simulink subsystem "serial_input_subsystem"  (R2020a)
settings: Solver=VariableStepAuto  StartTime=0.0  StopTime=10.0  RelTol=1e-3
libraries: frdmk64flib x2
settings Model: Creator=Ethan  LastModifiedBy=Ethan

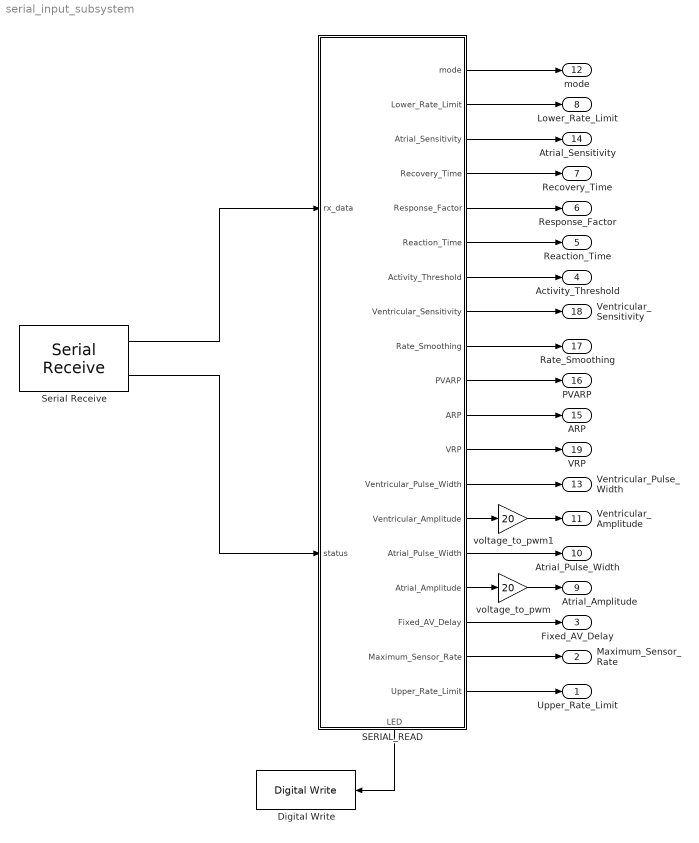
== system serial_input_subsystem ==
  Digital Write : frdmk64flib/Digital Write  Whichpin=BLUE_LED
  SERIAL_READ : Stateflow chart  TreatAsAtomicUnit=on
      settings: PortSchema="{\"entries\":[{\"content\":{\"sides\":[{\"content\":{\"connectorIds\":[\"In2\",\"In1\"]},\"type\":\"ConnectorPlacement.EquallySpacedRectSide\",\"uuid\":\"7925fb1d-c012-46b4-a76b-df094bb3995e\"},{\"content\":{\"connectorIds\":[\"Out1\",\"Out2\",\"Out3\",\"Out4\",\"Out5\",\"Out6\",\"Out7\",\"Out8\",\"Out9\",\"Out10\",\"Out11\",\"Out12\",\"Out13\",\"Out14\",\"Out15\",\"Out16\",\"Out18\",\"Out20\",\"Out19\"],\"side\":\"RIGHT\"},\"type\":\"ConnectorPlacement.EquallySpacedRectSide\",\"uuid\":\"8182b149-1b25-42ed-a9c6-d652f0475bdf\"},{\"content\":{\"connectorIds\":[\"Out17\"],\"side\":\"TOP\"},\"type\":\"ConnectorPlacement.EquallySpacedRectSide\",\"uuid\":\"014ecb25-725b-45bf-b2bd-0487c3cb83c8\"}]},\"type\":\"ConnectorPlacement.EquallySpacedConnector\",\"uuid\":\"b7c7ca09-4347-41ae-aa03-be4e7decd789\"}],\"packageUris\":[\"http://schema.mathworks.com/mf0/Connector/19700101\"],\"version\":\"1.0\"}"
  Serial Receive : frdmk64flib/Serial Receive  SCIModule=0  Baudrate=uint32(9600)  Parity=None  StopBits=1  HardwareFlowControl=None  ByteOrder=LittleEndian  DataType=uint8  DataLength=66  BlockingMode=off  OutputStatus=on  SampleTime=-1
  voltage_to_pwm : Gain  Gain=20  OutDataTypeStr=Inherit: Same as input
  voltage_to_pwm1 : Gain  Gain=20  OutDataTypeStr=Inherit: Same as input
  Upper_Rate_Limit : Outport
  Maximum_Sensor_Rate : Outport  Port=2
  Fixed_AV_Delay : Outport  Port=3
  Activity_Threshold : Outport  Port=4
  Reaction_Time : Outport  Port=5
  Response_Factor : Outport  Port=6
  Recovery_Time : Outport  Port=7
  Lower_Rate_Limit : Outport  Port=8
  Atrial_Amplitude : Outport  Port=9
  Atrial_Pulse_Width : Outport  Port=10
  Ventricular_Amplitude : Outport  Port=11
  mode : Outport  Port=12
  Ventricular_Pulse_Width : Outport  Port=13
  Atrial_Sensitivity : Outport  Port=14
  ARP : Outport  Port=15
  PVARP : Outport  Port=16
  Rate_Smoothing : Outport  Port=17
  Ventricular_Sensitivity : Outport  Port=18
  VRP : Outport  Port=19
  wires:
  voltage_to_pwm/1 -> Atrial_Amplitude/1
  SERIAL_READ/8(VRP) -> VRP/1
  SERIAL_READ/17(LED) -> Digital Write/1
  SERIAL_READ/2(Maximum_Sensor_Rate) -> Maximum_Sensor_Rate/1
  SERIAL_READ/12(Ventricular_Sensitivity) -> Ventricular_Sensitivity/1
  Serial Receive/2 -> SERIAL_READ/2(status)
  SERIAL_READ/3(Fixed_AV_Delay) -> Fixed_AV_Delay/1
  SERIAL_READ/9(ARP) -> ARP/1
  Serial Receive/1 -> SERIAL_READ/1(rx_data)
  SERIAL_READ/6(Ventricular_Amplitude) -> voltage_to_pwm1/1
  SERIAL_READ/14(Reaction_Time) -> Reaction_Time/1
  SERIAL_READ/4(Atrial_Amplitude) -> voltage_to_pwm/1
  SERIAL_READ/16(Recovery_Time) -> Recovery_Time/1
  SERIAL_READ/7(Ventricular_Pulse_Width) -> Ventricular_Pulse_Width/1
  SERIAL_READ/19(mode) -> mode/1
  SERIAL_READ/1(Upper_Rate_Limit) -> Upper_Rate_Limit/1
  voltage_to_pwm1/1 -> Ventricular_Amplitude/1
  SERIAL_READ/11(Rate_Smoothing) -> Rate_Smoothing/1
  SERIAL_READ/10(PVARP) -> PVARP/1
  SERIAL_READ/18(Atrial_Sensitivity) -> Atrial_Sensitivity/1
  SERIAL_READ/20(Lower_Rate_Limit) -> Lower_Rate_Limit/1
  SERIAL_READ/5(Atrial_Pulse_Width) -> Atrial_Pulse_Width/1
  SERIAL_READ/15(Response_Factor) -> Response_Factor/1
  SERIAL_READ/13(Activity_Threshold) -> Activity_Threshold/1

== stateflow chart serial_input_subsystem/SERIAL_READ ==
  state ASSIGN_VALUES
    entry:
    mode = rx_data(1);
    Lower_Rate_Limit_BYTE = rx_data(2);
    Lower_Rate_Limit = uint16(Lower_Rate_Limit_BYTE);
    Upper_Rate_Limit = rx_data(3);
    Maximum_Sensor_Rate = typecast(rx_data(4:5), 'uint16');
    Fixed_AV_Delay = typecast(rx_data(6:7), 'uint16');
    Atrial_Amplitude = typecast(rx_data(8:15), 'double');
    Atrial_Pulse_Width = typecast(rx_data(16:23), 'double');
    Ventricular_Amplitude = typecast(rx_data(24:31), 'double');
    Ventricular_Pulse_Width = typecast(rx_data(32:39), 'double');
    Atrial_Sensitivity = typecast(rx_data(40:47), 'double');
    VRP = typecast(rx_data(48:49), 'uint16');
    ARP = typecast(rx_data(50:51), 'uint16');
    PVARP = typecast(rx_data(52:53), 'uint16');
    Rate_Smoothing = rx_data(54);
    Ventricular_Sensitivity = typecast(rx_data(55:62), 'double');
    Activity_Threshold = rx_data(63);
    Reaction_Time = rx_data(64);
    Response_Factor = rx_data(65);
    Recovery_Time = rx_data(66);
  state INITIAL
    entry:
    mode = 0;
    Lower_Rate_Limit = 0;
    Upper_Rate_Limit = 0;
    Maximum_Sensor_Rate = 0;
    Fixed_AV_Delay = 0;
    Atrial_Amplitude = 0;
    Atrial_Pulse_Width = 0;
    Ventricular_Amplitude = 0;
    Ventricular_Pulse_Width = 0;
    Atrial_Sensitivity = 0;
    VRP = 0;
    ARP = 0;
    PVARP = 0;
    Rate_Smoothing = 0;
    Ventricular_Sensitivity = 0;
    Activity_Threshold = 0;
    Reaction_Time = 0;
    Response_Factor = 0;
    Recovery_Time = 0;
    LED = 0;
  state STANDBY
    entry:
    LED = 0;
  state LED_ACK
    entry:
    LED = 1;
  (default) -> INITIAL
  STANDBY -> ASSIGN_VALUES : [status == 0]
  INITIAL -> STANDBY
  LED_ACK -> STANDBY : [after(200,msec)]
  ASSIGN_VALUES -> LED_ACK
  data: rx_data input uint8; status input uint8; Upper_Rate_Limit output uint8; Maximum_Sensor_Rate output uint16; Fixed_AV_Delay output uint16; Atrial_Amplitude output double; Atrial_Pulse_Width output double; Ventricular_Amplitude output double; Ventricular_Pulse_Width output double; VRP output uint16; ARP output uint16; PVARP output uint16; Rate_Smoothing output uint8; Ventricular_Sensitivity output double; Activity_Threshold output uint8; Reaction_Time output uint8; Response_Factor output uint8; Recovery_Time output uint8; LED output; Atrial_Sensitivity output double; mode output uint8; Lower_Rate_Limit output uint16; Lower_Rate_Limit_BYTE local uint8
